simulink model "OurSetup"  (Simulink 8.8)
settings: Solver=ode45  StartTime=0.0  StopTime=20  RelTol=1e-3  EnableMultiTasking=on
undefined symbols (not defined in the file): h
libraries: simulink x1
settings Model: Creator=rbabuska  LastModifiedBy=ojacobs
settings OptimizationCC: ExpressionDepthLimit=2147483647  InitFltsAndDblsToZero=on
settings DebuggingCC: SaveWithParameterizedLinksMsg=none  SignalResolutionControl=TryResolveAllWithWarning  SolverPrmCheckMsg=warning  MultiTaskCondExecSysMsg=none
settings GRTTargetCC: TargetFcnLib=ansi_tfl_tmw.mat

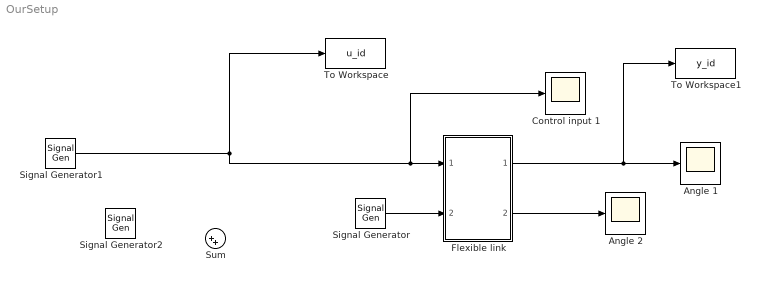
== system OurSetup ==
  Angle 1 : Scope
  Angle 2 : Scope
  Control input 1 : Scope
  Flexible link : Subsystem  mask{Ts=h}
      mask prompts: Ts "Sampling period"
      mask Display: disp('Flexible link')
  Signal Generator : SignalGenerator  Amplitude=0  Frequency=2
  Signal Generator1 : SignalGenerator  Amplitude=.5  Frequency=0.5
  Signal Generator2 : SignalGenerator  Amplitude=.2  Frequency=0.9
  Sum : Sum  Inputs=|++
  To Workspace : ToWorkspace  VariableName=u_id  SampleTime=-1
  To Workspace1 : ToWorkspace  VariableName=y_id  SampleTime=-1
  wires:
  Signal Generator1/1 -> Flexible link/1(Input 1), Control input 1/1, To Workspace/1
  Flexible link/1(Angle 1) -> To Workspace1/1, Angle 1/1
  Flexible link/2(Angle 2) -> Angle 2/1
  Signal Generator/1 -> Flexible link/2(Input 2)

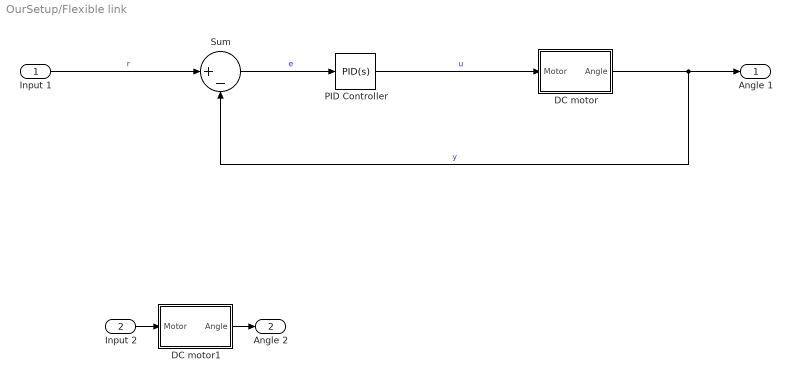
== system OurSetup/Flexible link ==
  Input 1 : Inport
  Input 2 : Inport  Port=2
  DC motor : Subsystem  mask{h=Ts, setupnr=1}
      mask prompts: h "Sample time [s]:"; setupnr "Setup number (for instance 1 or 2, etc.)"
      mask Display: disp('DC Motor')
  DC motor1 : Subsystem  mask{h=Ts, setupnr=2}
      mask prompts: h "Sample time [s]:"; setupnr "Setup number (for instance 1 or 2, etc.)"
      mask Display: disp('DC Motor')
  PID Controller : simulink/Continuous/PID Controller  Controller=PID  TimeDomain=Continuous-time  SampleTime=-1  IntegratorMethod=Forward Euler  FilterMethod=Forward Euler  Form=Parallel  UseFilter=on  ControllerParametersSource=internal  P=1  I=0.5  D=0  N=10  InitialConditionSource=internal  InitialConditionForIntegrator=0  InitialConditionForFilter=0  ExternalReset=none  LimitOutput=off  UpperSaturationLimit=inf  LowerSaturationLimit=-inf  LinearizeAsGain=on  AntiWindupMode=none  Kb=1  TrackingMode=off  Kt=1  PParamMin=[]  PParamMax=[]  IParamMin=[]  IParamMax=[]  DParamMin=[]  DParamMax=[]  NParamMin=[]  NParamMax=[]  KbParamMin=[]  KbParamMax=[]  KtParamMin=[]  KtParamMax=[]  POutMin=[]  POutMax=[]  IOutMin=[]  IOutMax=[]  DOutMin=[]  DOutMax=[]  NOutMin=[]  NOutMax=[]  KbOutMin=[]  KbOutMax=[]  KtOutMin=[]  KtOutMax=[]  IntegratorOutMin=[]  IntegratorOutMax=[]  FilterOutMin=[]  FilterOutMax=[]  SumOutMin=[]  SumOutMax=[]  SumI1OutMin=[]  SumI1OutMax=[]  SumI2OutMin=[]  SumI2OutMax=[]  SumI3OutMin=[]  SumI3OutMax=[]  SumDOutMin=[]  SumDOutMax=[]  SaturationOutMin=[]  SaturationOutMax=[]  IntegratorContinuousStateAttributes=''  IntegratorStateMustResolveToSignalObject=off  IntegratorRTWStateStorageClass=Auto  FilterContinuousStateAttributes=''  FilterStateMustResolveToSignalObject=off  FilterRTWStateStorageClass=Auto  DifferentiatorICPrevScaledInput=0  DifferentiatorOutMin=[]  DifferentiatorOutMax=[]
  Sum : Sum  Inputs=|+-
  Angle 1 : Outport
  Angle 2 : Outport  Port=2
  wires:
  Input 1/1 -> Sum/1  "r"
  DC motor/1(Angle) -> Sum/2, Angle 1/1  "y"
  Input 2/1 -> DC motor1/1(Motor)
  DC motor1/1(Angle) -> Angle 2/1
  Sum/1 -> PID Controller/1  "e"
  PID Controller/1 -> DC motor/1(Motor)  "u"

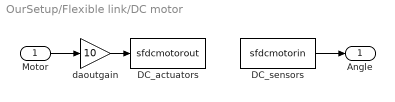
== system OurSetup/Flexible link/DC motor ==
  Motor : Inport
  DC_actuators : S-Function  FunctionName=sfdcmotorout  Parameters=Ts, H  SFunctionDeploymentMode=off  EnableBusSupport=off  mask(Serial Out){Ts=h, setupnr=setupnr}
      mask prompts: Ts "Sample time:"; setupnr "Setup number:"
      mask help: Serial line output block
      mask init:
      | H=fugiboard('Open', ['mops' num2str(setupnr)]);
      mask Help: Serial Out block is designed as a serial communication output block for real time data acquisition, signal processing and control applications.
      mask Display: disp('DC Motor');
  DC_sensors : S-Function  FunctionName=sfdcmotorin  Parameters=Ts, H  SFunctionDeploymentMode=off  EnableBusSupport=off  mask(Serial Out){Ts=h, setupnr=setupnr}
      mask prompts: Ts "Sample time:"; setupnr "Setup number"
      mask help: Serial line output block
      mask init:
      | H=fugiboard('Open', ['mops' num2str(setupnr)]);
      mask Help: Serial Out block is designed as a serial communication output block for real time data acquisition, signal processing and control applications.
      mask Display: disp('DC Motor');
  daoutgain : Gain  Gain=10  SaturateOnIntegerOverflow=on  OutDataTypeStr=Inherit: Same as input  ParamDataTypeStr=Inherit: Same as input
  Angle : Outport
  wires:
  Motor/1 -> daoutgain/1
  DC_sensors/1 -> Angle/1
  daoutgain/1 -> DC_actuators/1

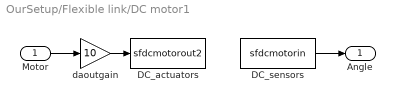
== system OurSetup/Flexible link/DC motor1 ==
  Motor : Inport
  DC_actuators : S-Function  FunctionName=sfdcmotorout2  Parameters=Ts, H  SFunctionDeploymentMode=off  EnableBusSupport=off  mask(Serial Out){Ts=h, setupnr=setupnr}
      mask prompts: Ts "Sample time:"; setupnr "Setup number:"
      mask help: Serial line output block
      mask init:
      | H=fugiboard('Open', ['mops' num2str(setupnr)]);
      mask Help: Serial Out block is designed as a serial communication output block for real time data acquisition, signal processing and control applications.
      mask Display: disp('DC Motor');
  DC_sensors : S-Function  FunctionName=sfdcmotorin  Parameters=Ts, H  SFunctionDeploymentMode=off  EnableBusSupport=off  mask(Serial Out){Ts=h, setupnr=setupnr}
      mask prompts: Ts "Sample time:"; setupnr "Setup number"
      mask help: Serial line output block
      mask init:
      | H=fugiboard('Open', ['mops' num2str(setupnr)]);
      mask Help: Serial Out block is designed as a serial communication output block for real time data acquisition, signal processing and control applications.
      mask Display: disp('DC Motor');
  daoutgain : Gain  Gain=10  SaturateOnIntegerOverflow=on  OutDataTypeStr=Inherit: Same as input  ParamDataTypeStr=Inherit: Same as input
  Angle : Outport
  wires:
  daoutgain/1 -> DC_actuators/1
  DC_sensors/1 -> Angle/1
  Motor/1 -> daoutgain/1
